simulink model "IEEE_9bus_new_o"  (R2024a)
settings: Solver=ode45  StartTime=0.0  StopTime=60/60  RelTol=1e-3  EnableMultiTasking=on
PreLoadFcn:
  | faultType = "ABCG";
  | faultLineStr = "Line 7-8";
  | faultDistance = 50;
  | L78_Length = 50;
  | L89_Length = 50;
  | L96_Length = 50;
  | L64_Length = 50;
  | L45_Length = 50;
  | L57_Length = 50;
  | 
  | mdl = load('lineIdentificationModel.mat');
  | lineMdl = mdl.treeModel;
  | 
  | mdl = load('typeIdentificationModelV2.mat');
  | typeMdl = mdl.treeModel;
  | 
  | mdl = load('faultLocationModel.mat');
  | locationMdl = mdl.treeModel;
libraries: dspstat3 x36, simulink x24, spsThreePhasePISectionLineLib x12, spsThreePhaseVIMeasurementLib x12, spsLoadFlowBusLib x9, spsThreePhaseFaultLib x6, jailib x3, spsThreePhaseSourceLib x3, spsThreePhaseTransformerTwoWindingsLib x3, statsLibrary x3, spsThreePhaseBreakerLib x3, sps_lib x1
(part 2 of 3)

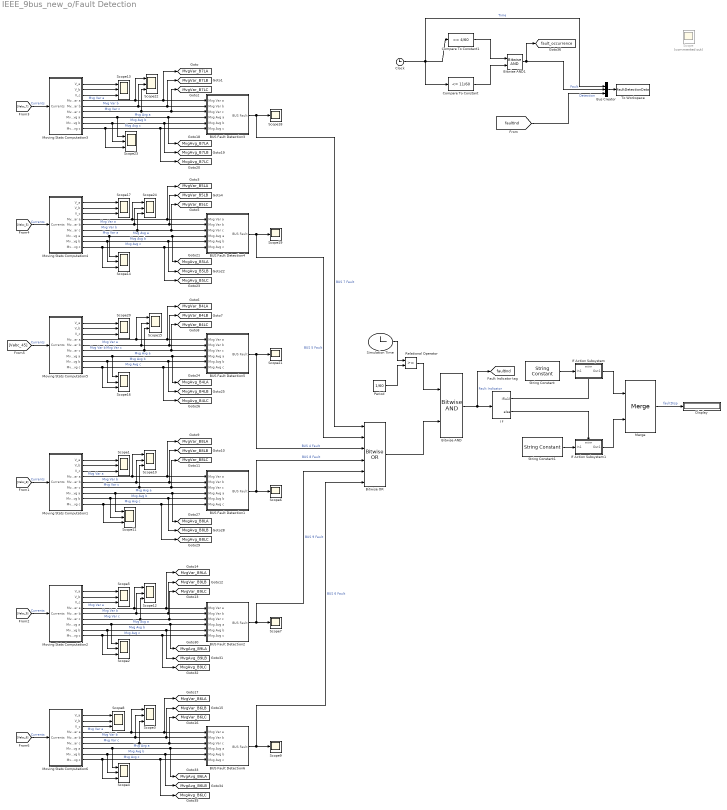
== system IEEE_9bus_new_o/Fault Detection ==
  BUS Fault Detection1 : Subsystem
  BUS Fault Detection2 : Subsystem
  BUS Fault Detection3 : Subsystem
  BUS Fault Detection4 : Subsystem
  BUS Fault Detection5 : Subsystem
  BUS Fault Detection6 : Subsystem
  Bitwise AND : simulink/Logic and Bit Operations/Bitwise Operator  logicop=AND  UseBitMask=off  NumInputPorts=2  BitMask=bin2dec('11011001')  BitMaskRealWorld=Stored Integer
      settings: LibrarySourceBlock=|
      | simulink/Quick Insert/Logic and Bit
      | Operations/Bitwise AND
  Bitwise AND1 : simulink/Logic and Bit Operations/Bitwise Operator  logicop=AND  UseBitMask=off  NumInputPorts=2  BitMask=bin2dec('11011001')  BitMaskRealWorld=Stored Integer
      settings: LibrarySourceBlock=|
      | simulink/Quick Insert/Logic and Bit
      | Operations/Bitwise AND
  Bitwise OR : simulink/Logic and Bit Operations/Bitwise Operator  logicop=OR  UseBitMask=off  NumInputPorts=6  BitMask=bin2dec('11011001')  BitMaskRealWorld=Stored Integer
      settings: LibrarySourceBlock=|
      | simulink/Quick Insert/Logic and Bit
      | Operations/Bitwise OR
  Bus Creator : BusCreator  Inputs=3
  Clock : Clock
  Compare To Constant : simulink/Logic and Bit Operations/Compare To Constant  relop=<=  const=11/60  OutDataTypeStr=boolean
  Compare To Constant1 : simulink/Logic and Bit Operations/Compare To Constant  relop=>=  const=4/60  OutDataTypeStr=boolean
  Display : Display
  I f : If  IfExpression=u1
  If Action Subsystem : Subsystem  TreatAsAtomicUnit=on
  If Action Subsystem1 : Subsystem  TreatAsAtomicUnit=on
  Merge : Merge
  Moving Stats Computation1 : Subsystem
  Moving Stats Computation2 : Subsystem
  Moving Stats Computation3 : Subsystem
  Moving Stats Computation4 : Subsystem
  Moving Stats Computation5 : Subsystem
  Moving Stats Computation6 : Subsystem
  Period : Constant  Value=1/60
  Relational Operator : RelationalOperator  OutDataTypeStr=boolean  RndMeth=Simplest  InputSameDT=off
  Scope : Scope  Commented=on  NumInputPorts=2
  Scope{1..5,8,10..17,20,22..24} (18 alike) : Scope  NumInputPorts=3
  Scope{6..7,9,18..19,21} (6 alike) : Scope
  Simulation Time : Clock
  String Constant : StringConstant  String="\"Faulted\""
  String Constant1 : StringConstant  String="\"\""
  To Workspace : ToWorkspace  VariableName=faultDetectionData  SaveFormat=Timeseries  SampleTime=-1
  tag scope: MvgAvg_B4LA=global, MvgAvg_B4LB=global, MvgAvg_B4LC=global, MvgAvg_B5LA=global, MvgAvg_B5LB=global, MvgAvg_B5LC=global, MvgAvg_B6LA=global, MvgAvg_B6LB=global, MvgAvg_B6LC=global, MvgAvg_B7LA=global, MvgAvg_B7LB=global, MvgAvg_B7LC=global, MvgAvg_B8LA=global, MvgAvg_B8LB=global, MvgAvg_B8LC=global, MvgAvg_B9LA=global, MvgAvg_B9LB=global, MvgAvg_B9LC=global, MvgVar_B4LA=global, MvgVar_B4LB=global, MvgVar_B4LC=global, MvgVar_B5LA=global, MvgVar_B5LB=global, MvgVar_B5LC=global, MvgVar_B6LA=global, MvgVar_B6LB=global, MvgVar_B6LC=global, MvgVar_B7LA=global, MvgVar_B7LB=global, MvgVar_B7LC=global, MvgVar_B8LA=global, MvgVar_B8LB=global, MvgVar_B8LC=global, MvgVar_B9LA=global, MvgVar_B9LB=global, MvgVar_B9LC=global, faultInd=global, fault_occurrence=global
  wires:
  BUS Fault Detection5/1(BUS Fault) -> Bitwise OR/3, Scope21/1  "BUS 4 Fault"
  BUS Fault Detection3/1(BUS Fault) -> Scope18/1, Bitwise OR/1  "BUS 7 Fault"
  Moving Stats Computation2/3(V_c) -> Scope5/3
  Moving Stats Computation6/5(Mvg Var b) -> BUS Fault Detection6/2(Mvg Var b), [MvgVar_B6LB], Scope3/2  "Mvg Var b"
  Moving Stats Computation6/7(Mvg Avg a) -> BUS Fault Detection6/4(Mvg Avg a), [MvgAvg_B6LA], Scope4/1  "Mvg Avg a"
  Moving Stats Computation3/6(Mvg Var c) -> BUS Fault Detection3/3(Mvg Var c), [MvgVar_B7LC], Scope22/3  "Mvg Var c"
  BUS Fault Detection6/1(BUS Fault) -> Bitwise OR/6, Scope9/1  "BUS 6 Fault"
  Moving Stats Computation1/8(Mvg Avg b) -> BUS Fault Detection1/5(Mvg Avg b), [MvgAvg_B8LB], Scope11/2  "Mvg Avg b"
  Moving Stats Computation5/4(Mvg Var a) -> BUS Fault Detection5/1(Mvg Var a), [MvgVar_B4LA], Scope15/1  "Mvg Var a"
  Moving Stats Computation1/5(Mvg Var b) -> BUS Fault Detection1/2(Mvg Var b), [MvgVar_B8LB], Scope10/2  "Mvg Var b"
  [Vabc_9] -> Moving Stats Computation2/1(Currents)  "Currents"
  Moving Stats Computation4/9(Mvg Avg c) -> BUS Fault Detection4/6(Mvg Avg c), [MvgAvg_B5LC], Scope14/3  "Mvg Avg c"
  Moving Stats Computation3/5(Mvg Var b) -> [MvgVar_B7LB], BUS Fault Detection3/2(Mvg Var b), Scope22/2  "Mvg Var b"
  Moving Stats Computation1/2(V_b) -> Scope1/2
  Moving Stats Computation1/7(Mvg Avg a) -> BUS Fault Detection1/4(Mvg Avg a), [MvgAvg_B8LA], Scope11/1  "Mvg Avg a"
  [Vabc_7] -> Moving Stats Computation3/1(Currents)  "Currents"
  Moving Stats Computation5/6(Mvg Var c) -> BUS Fault Detection5/3(Mvg Var c), [MvgVar_B4LC], Scope15/3  "Mvg Var c"
  Moving Stats Computation2/7(Mvg Avg a) -> BUS Fault Detection2/4(Mvg Avg a), [MvgAvg_B9LA], Scope2/1  "Mvg Avg a"
  Moving Stats Computation5/9(Mvg Avg c) -> BUS Fault Detection5/6(Mvg Avg c), [MvgAvg_B4LC], Scope16/3  "Mvg Avg c"
  Moving Stats Computation2/2(V_b) -> Scope5/2
  Moving Stats Computation4/1(V_a) -> Scope17/1
  Moving Stats Computation5/2(V_b) -> Scope20/2
  Moving Stats Computation3/1(V_a) -> Scope13/1
  Moving Stats Computation5/7(Mvg Avg a) -> BUS Fault Detection5/4(Mvg Avg a), [MvgAvg_B4LA], Scope16/1  "Mvg Avg a"
  [Vabc_8] -> Moving Stats Computation1/1(Currents)  "Currents"
  Moving Stats Computation6/2(V_b) -> Scope8/2
  Moving Stats Computation5/5(Mvg Var b) -> BUS Fault Detection5/2(Mvg Var b), [MvgVar_B4LB], Scope15/2  "Mvg Var b"
  Moving Stats Computation1/1(V_a) -> Scope1/1
  Moving Stats Computation5/8(Mvg Avg b) -> BUS Fault Detection5/5(Mvg Avg b), [MvgAvg_B4LB], Scope16/2  "Mvg Avg b"
  Moving Stats Computation2/1(V_a) -> Scope5/1
  Moving Stats Computation4/8(Mvg Avg b) -> BUS Fault Detection4/5(Mvg Avg b), [MvgAvg_B5LB], Scope14/2  "Mvg Avg b"
  BUS Fault Detection4/1(BUS Fault) -> Scope19/1, Bitwise OR/2  "BUS 5 Fault"
  BUS Fault Detection1/1(BUS Fault) -> Scope6/1, Bitwise OR/4  "BUS 8 Fault"
  Moving Stats Computation6/9(Mvg Avg c) -> BUS Fault Detection6/6(Mvg Avg c), [MvgAvg_B6LC], Scope4/3  "Mvg Avg c"
  Moving Stats Computation3/9(Mvg Avg c) -> [MvgAvg_B7LC], BUS Fault Detection3/6(Mvg Avg c), Scope23/3  "Mvg Avg c"
  Moving Stats Computation4/3(V_c) -> Scope17/3
  [Vabc_5] -> Moving Stats Computation4/1(Currents)  "Currents"
  Moving Stats Computation6/1(V_a) -> Scope8/1
  Moving Stats Computation5/1(V_a) -> Scope20/1
  Moving Stats Computation1/3(V_c) -> Scope1/3
  Moving Stats Computation2/5(Mvg Var b) -> BUS Fault Detection2/2(Mvg Var b), [MvgVar_B9LB], Scope12/2  "Mvg Var b"
  Moving Stats Computation5/3(V_c) -> Scope20/3
  Moving Stats Computation6/3(V_c) -> Scope8/3
  Moving Stats Computation3/8(Mvg Avg b) -> [MvgAvg_B7LB], BUS Fault Detection3/5(Mvg Avg b), Scope23/2  "Mvg Avg b"
  [Vabc_45] -> Moving Stats Computation5/1(Currents)  "Currents"
  Moving Stats Computation3/3(V_c) -> Scope13/3
  Moving Stats Computation6/8(Mvg Avg b) -> BUS Fault Detection6/5(Mvg Avg b), [MvgAvg_B6LB], Scope4/2  "Mvg Avg b"
  Moving Stats Computation4/7(Mvg Avg a) -> BUS Fault Detection4/4(Mvg Avg a), [MvgAvg_B5LA], Scope14/1  "Mvg Avg a"
  Moving Stats Computation3/7(Mvg Avg a) -> BUS Fault Detection3/4(Mvg Avg a), [MvgAvg_B7LA], Scope23/1  "Mvg Avg a"
  Moving Stats Computation3/4(Mvg Var a) -> [MvgVar_B7LA], BUS Fault Detection3/1(Mvg Var a), Scope22/1  "Mvg Var a"
  Moving Stats Computation2/6(Mvg Var c) -> BUS Fault Detection2/3(Mvg Var c), [MvgVar_B9LC], Scope12/3  "Mvg Var c"
  Moving Stats Computation3/2(V_b) -> Scope13/2
  Moving Stats Computation2/9(Mvg Avg c) -> BUS Fault Detection2/6(Mvg Avg c), [MvgAvg_B9LC], Scope2/3  "Mvg Avg c"
  Moving Stats Computation4/2(V_b) -> Scope17/2
  Moving Stats Computation6/6(Mvg Var c) -> BUS Fault Detection6/3(Mvg Var c), [MvgVar_B6LC], Scope3/3  "Mvg Var c"
  Moving Stats Computation6/4(Mvg Var a) -> BUS Fault Detection6/1(Mvg Var a), [MvgVar_B6LA], Scope3/1  "Mvg Var a"
  BUS Fault Detection2/1(BUS Fault) -> Scope7/1, Bitwise OR/5  "BUS 9 Fault"
  Moving Stats Computation2/8(Mvg Avg b) -> BUS Fault Detection2/5(Mvg Avg b), [MvgAvg_B9LB], Scope2/2  "Mvg Avg b"
  Moving Stats Computation2/4(Mvg Var a) -> BUS Fault Detection2/1(Mvg Var a), [MvgVar_B9LA], Scope12/1  "Mvg Var a"
  [Vabc_6] -> Moving Stats Computation6/1(Currents)  "Currents"
  Moving Stats Computation1/9(Mvg Avg c) -> BUS Fault Detection1/6(Mvg Avg c), [MvgAvg_B8LC], Scope11/3  "Mvg Avg c"
  Moving Stats Computation1/4(Mvg Var a) -> BUS Fault Detection1/1(Mvg Var a), [MvgVar_B8LA], Scope10/1  "Mvg Var a"
  Moving Stats Computation1/6(Mvg Var c) -> BUS Fault Detection1/3(Mvg Var c), [MvgVar_B8LC], Scope10/3  "Mvg Var c"
  Simulation Time/1 -> Relational Operator/1
  Period/1 -> Relational Operator/2
  Relational Operator/1 -> Bitwise AND/1
  Bitwise OR/1 -> Bitwise AND/2
  Bitwise AND/1 -> [faultInd], I f/1  "Fault Indicator"
  I f/1 -> If Action Subsystem/Action
  I f/2 -> If Action Subsystem1/Action
  String Constant/1 -> If Action Subsystem/1(In1)
  String Constant1/1 -> If Action Subsystem1/1(In1)
  If Action Subsystem/1(Out1) -> Merge/1
  If Action Subsystem1/1(Out1) -> Merge/2
  Moving Stats Computation4/4(Mvg Var a) -> BUS Fault Detection4/1(Mvg Var a), [MvgVar_B5LA], Scope24/1  "Mvg Var a"
  Moving Stats Computation4/5(Mvg Var b) -> BUS Fault Detection4/2(Mvg Var b), [MvgVar_B5LB], Scope24/2  "Mvg Var b"
  Moving Stats Computation4/6(Mvg Var c) -> BUS Fault Detection4/3(Mvg Var c), [MvgVar_B5LC], Scope24/3  "Mvg Var a"
  Merge/1 -> Display/1  "faultDisp"
  Clock/1 -> Bus Creator/1, Compare To Constant1/1, Compare To Constant/1  "Time"
  Compare To Constant1/1 -> Bitwise AND1/1
  Compare To Constant/1 -> Bitwise AND1/2
  Bitwise AND1/1 -> Bus Creator/2, [fault_occurrence]  "Fault"
  [faultInd] -> Bus Creator/3  "Detection"
  Bus Creator/1 -> To Workspace/1

== system IEEE_9bus_new_o/Fault Line Identification ==
  Display : Display
  Fault Line Prediction : statsLibrary/Classification/ClassificationTree Predict  TrainedLearner=lineMdl  ShowOutputScore=off  LabelOutMin=[]  LabelOutMax=[]  ScoreOutMin=[]  ScoreOutMax=[]  RawScoreOutMin=[]  RawScoreOutMax=[]  StoredEnumName=lineMdl_enumLabels
  If : If  IfExpression=u1~=0
  If Action Subsystem : Subsystem  TreatAsAtomicUnit=on
  If Action Subsystem1 : Subsystem  TreatAsAtomicUnit=on
  Merge : Merge
  String Constant : StringConstant  String="\"\""
  To String : ToString
  wires:
  If Action Subsystem/1(Out1) -> Merge/1
  String Constant/1 -> If Action Subsystem1/1(In1)
  If/2 -> If Action Subsystem1/Action
  If Action Subsystem1/1(Out1) -> Merge/2
  To String/1 -> If Action Subsystem/1(In1)
  [faultInd] -> If/1
  [MvgStats] -> Fault Line Prediction/1
  Fault Line Prediction/1 -> To String/1
  If/1 -> If Action Subsystem/Action
  Merge/1 -> Display/1  "LineDisp"

== system IEEE_9bus_new_o/Fault Location ==
  Display : Display
  Fault Location Prediction : statsLibrary/Regression/RegressionTree Predict  TrainedLearner=locationMdl  OutMin=[]  OutMax=[]
  If : If  IfExpression=u1~=0
  If Action Subsystem : Subsystem  TreatAsAtomicUnit=on
  If Action Subsystem1 : Subsystem  TreatAsAtomicUnit=on
  Merge : Merge
  String Constant : StringConstant  String="\"\""
  To String : ToString
  wires:
  If Action Subsystem/1(Out1) -> Merge/1
  String Constant/1 -> If Action Subsystem1/1(In1)
  If/2 -> If Action Subsystem1/Action
  If Action Subsystem1/1(Out1) -> Merge/2
  To String/1 -> If Action Subsystem/1(In1)
  [faultInd] -> If/1
  [MvgStats] -> Fault Location Prediction/1
  Fault Location Prediction/1 -> To String/1
  If/1 -> If Action Subsystem/Action
  Merge/1 -> Display/1  "LocationDisp"

== system IEEE_9bus_new_o/Fault Type Identification ==
  Display : Display
  Fault Type Prediction : statsLibrary/Classification/ClassificationTree Predict  TrainedLearner=typeMdl  ShowOutputScore=off  LabelOutMin=[]  LabelOutMax=[]  ScoreOutMin=[]  ScoreOutMax=[]  RawScoreOutMin=[]  RawScoreOutMax=[]  StoredEnumName=typeMdl_enumLabels
  If : If  IfExpression=u1~=0
  If Action Subsystem : Subsystem  TreatAsAtomicUnit=on
  If Action Subsystem1 : Subsystem  TreatAsAtomicUnit=on
  Merge : Merge
  String Constant : StringConstant  String="\"\""
  To String : ToString
  wires:
  If/1 -> If Action Subsystem/Action
  Fault Type Prediction/1 -> To String/1
  [MvgStats] -> Fault Type Prediction/1
  [faultInd] -> If/1
  To String/1 -> If Action Subsystem/1(In1)
  If Action Subsystem1/1(Out1) -> Merge/2
  If/2 -> If Action Subsystem1/Action
  String Constant/1 -> If Action Subsystem1/1(In1)
  If Action Subsystem/1(Out1) -> Merge/1
  Merge/1 -> Display/1  "TypeDisp"

== system IEEE_9bus_new_o/Relay System ==
  Bitwise AND2 : simulink/Logic and Bit Operations/Bitwise Operator  logicop=AND  UseBitMask=off  NumInputPorts=10  BitMask=bin2dec('11011001')  BitMaskRealWorld=Stored Integer
      settings: LibrarySourceBlock=|
      | simulink/Quick Insert/Logic and Bit
      | Operations/Bitwise AND
  Delay : Delay  DelayLength=1
  Delay1 : Delay  DelayLength=3
  Delay2 : Delay  DelayLength=4
  Delay3 : Delay  DelayLength=5
  Delay4 : Delay  DelayLength=6
  Delay5 : Delay  DelayLength=7
  Delay6 : Delay  DelayLength=8
  Delay7 : Delay  DelayLength=9
  Delay8 : Delay  DelayLength=10
  Delay9 : Delay  DelayLength=10
  Scope : Scope  NumInputPorts=3
  tag scope: tripInd=global
  wires:
  Bitwise AND2/1 -> Scope/3, [tripInd]  "Relay Activation"
  [faultInd] -> Scope/2, Delay/1, Delay1/1, Delay2/1, Delay3/1, Delay4/1, Delay5/1, Delay6/1, Delay7/1, Delay9/1, Delay8/1  "Detection"
  Delay4/1 -> Bitwise AND2/5
  Delay1/1 -> Bitwise AND2/2
  Delay9/1 -> Bitwise AND2/10
  Delay5/1 -> Bitwise AND2/6
  Delay3/1 -> Bitwise AND2/4
  Delay8/1 -> Bitwise AND2/9
  Delay6/1 -> Bitwise AND2/7
  Delay2/1 -> Bitwise AND2/3
  Delay/1 -> Bitwise AND2/1
  Delay7/1 -> Bitwise AND2/8
  [fault_occurrence] -> Scope/1  "Fault"

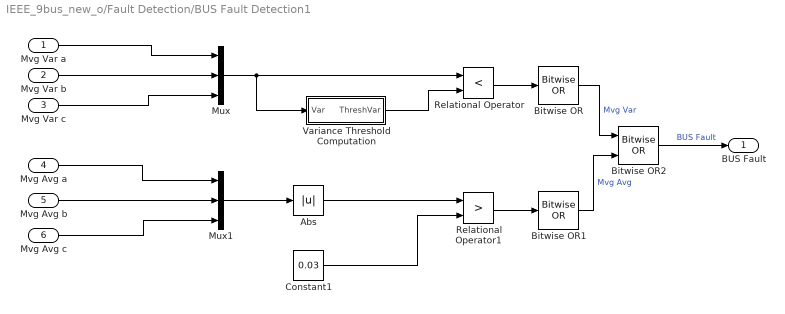
== system IEEE_9bus_new_o/Fault Detection/BUS Fault Detection1 ==
  Mvg Var a : Inport
  Mvg Var b : Inport  Port=2
  Mvg Var c : Inport  Port=3
  Mvg Avg a : Inport  Port=4
  Mvg Avg b : Inport  Port=5
  Mvg Avg c : Inport  Port=6
  Abs : Abs  SaturateOnIntegerOverflow=off
  Bitwise OR : simulink/Logic and Bit Operations/Bitwise Operator  logicop=OR  UseBitMask=off  BitMask=bin2dec('11011001')  BitMaskRealWorld=Stored Integer
      settings: LibrarySourceBlock=|
      | simulink/Quick Insert/Logic and Bit
      | Operations/Bitwise OR
  Bitwise OR1 : simulink/Logic and Bit Operations/Bitwise Operator  logicop=OR  UseBitMask=off  BitMask=bin2dec('11011001')  BitMaskRealWorld=Stored Integer
      settings: LibrarySourceBlock=|
      | simulink/Quick Insert/Logic and Bit
      | Operations/Bitwise OR
  Bitwise OR2 : simulink/Logic and Bit Operations/Bitwise Operator  logicop=OR  UseBitMask=off  NumInputPorts=2  BitMask=bin2dec('11011001')  BitMaskRealWorld=Stored Integer
      settings: LibrarySourceBlock=|
      | simulink/Quick Insert/Logic and Bit
      | Operations/Bitwise OR
  Constant1 : Constant  Value=0.03
  Mux : Mux  Inputs=3
  Mux1 : Mux  Inputs=3
  Relational Operator : RelationalOperator  Operator=<  OutDataTypeStr=boolean  RndMeth=Simplest  InputSameDT=off
  Relational Operator1 : RelationalOperator  Operator=>  OutDataTypeStr=boolean  RndMeth=Simplest  InputSameDT=off
  Variance Threshold Computation : Subsystem
  BUS Fault : Outport
  wires:
  Variance Threshold Computation/1(ThreshVar) -> Relational Operator/2
  Mvg Var b/1 -> Mux/2
  Abs/1 -> Relational Operator1/1
  Constant1/1 -> Relational Operator1/2
  Bitwise OR/1 -> Bitwise OR2/1  "Mvg Var"
  Bitwise OR1/1 -> Bitwise OR2/2  "Mvg Avg"
  Mux/1 -> Relational Operator/1, Variance Threshold Computation/1(Var)
  Relational Operator/1 -> Bitwise OR/1
  Bitwise OR2/1 -> BUS Fault/1  "BUS Fault"
  Relational Operator1/1 -> Bitwise OR1/1
  Mux1/1 -> Abs/1
  Mvg Avg a/1 -> Mux1/1
  Mvg Avg c/1 -> Mux1/3
  Mvg Var a/1 -> Mux/1
  Mvg Var c/1 -> Mux/3
  Mvg Avg b/1 -> Mux1/2

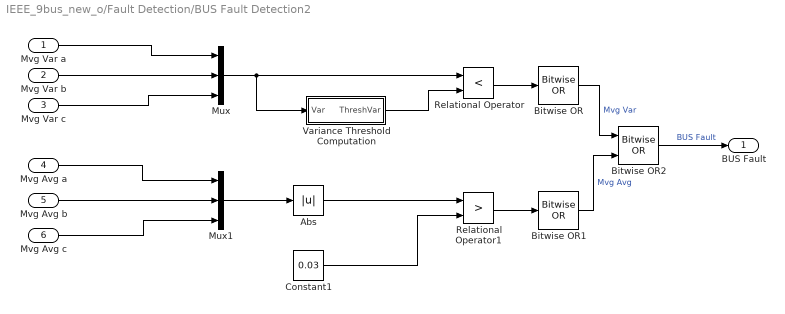
== system IEEE_9bus_new_o/Fault Detection/BUS Fault Detection2 ==
  Mvg Var a : Inport
  Mvg Var b : Inport  Port=2
  Mvg Var c : Inport  Port=3
  Mvg Avg a : Inport  Port=4
  Mvg Avg b : Inport  Port=5
  Mvg Avg c : Inport  Port=6
  Abs : Abs  SaturateOnIntegerOverflow=off
  Bitwise OR : simulink/Logic and Bit Operations/Bitwise Operator  logicop=OR  UseBitMask=off  BitMask=bin2dec('11011001')  BitMaskRealWorld=Stored Integer
      settings: LibrarySourceBlock=|
      | simulink/Quick Insert/Logic and Bit
      | Operations/Bitwise OR
  Bitwise OR1 : simulink/Logic and Bit Operations/Bitwise Operator  logicop=OR  UseBitMask=off  BitMask=bin2dec('11011001')  BitMaskRealWorld=Stored Integer
      settings: LibrarySourceBlock=|
      | simulink/Quick Insert/Logic and Bit
      | Operations/Bitwise OR
  Bitwise OR2 : simulink/Logic and Bit Operations/Bitwise Operator  logicop=OR  UseBitMask=off  NumInputPorts=2  BitMask=bin2dec('11011001')  BitMaskRealWorld=Stored Integer
      settings: LibrarySourceBlock=|
      | simulink/Quick Insert/Logic and Bit
      | Operations/Bitwise OR
  Constant1 : Constant  Value=0.03
  Mux : Mux  Inputs=3
  Mux1 : Mux  Inputs=3
  Relational Operator : RelationalOperator  Operator=<  OutDataTypeStr=boolean  RndMeth=Simplest  InputSameDT=off
  Relational Operator1 : RelationalOperator  Operator=>  OutDataTypeStr=boolean  RndMeth=Simplest  InputSameDT=off
  Variance Threshold Computation : Subsystem
  BUS Fault : Outport
  wires:
  Mvg Avg b/1 -> Mux1/2
  Mvg Var c/1 -> Mux/3
  Mvg Var a/1 -> Mux/1
  Mvg Avg c/1 -> Mux1/3
  Mvg Avg a/1 -> Mux1/1
  Mux1/1 -> Abs/1
  Relational Operator1/1 -> Bitwise OR1/1
  Bitwise OR2/1 -> BUS Fault/1  "BUS Fault"
  Relational Operator/1 -> Bitwise OR/1
  Mux/1 -> Variance Threshold Computation/1(Var), Relational Operator/1
  Bitwise OR1/1 -> Bitwise OR2/2  "Mvg Avg"
  Bitwise OR/1 -> Bitwise OR2/1  "Mvg Var"
  Constant1/1 -> Relational Operator1/2
  Abs/1 -> Relational Operator1/1
  Mvg Var b/1 -> Mux/2
  Variance Threshold Computation/1(ThreshVar) -> Relational Operator/2

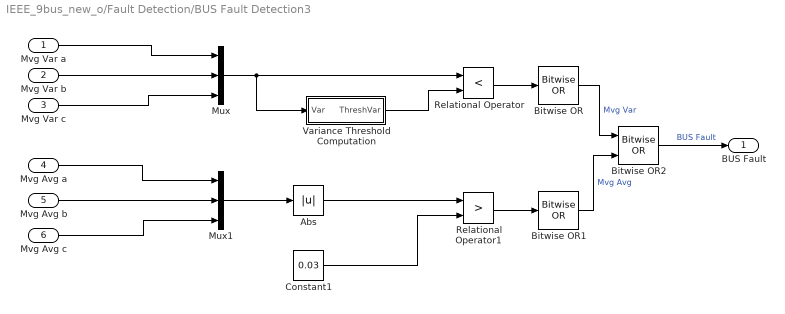
== system IEEE_9bus_new_o/Fault Detection/BUS Fault Detection3 ==
  Mvg Var a : Inport
  Mvg Var b : Inport  Port=2
  Mvg Var c : Inport  Port=3
  Mvg Avg a : Inport  Port=4
  Mvg Avg b : Inport  Port=5
  Mvg Avg c : Inport  Port=6
  Abs : Abs  SaturateOnIntegerOverflow=off
  Bitwise OR : simulink/Logic and Bit Operations/Bitwise Operator  logicop=OR  UseBitMask=off  BitMask=bin2dec('11011001')  BitMaskRealWorld=Stored Integer
      settings: LibrarySourceBlock=|
      | simulink/Quick Insert/Logic and Bit
      | Operations/Bitwise OR
  Bitwise OR1 : simulink/Logic and Bit Operations/Bitwise Operator  logicop=OR  UseBitMask=off  BitMask=bin2dec('11011001')  BitMaskRealWorld=Stored Integer
      settings: LibrarySourceBlock=|
      | simulink/Quick Insert/Logic and Bit
      | Operations/Bitwise OR
  Bitwise OR2 : simulink/Logic and Bit Operations/Bitwise Operator  logicop=OR  UseBitMask=off  NumInputPorts=2  BitMask=bin2dec('11011001')  BitMaskRealWorld=Stored Integer
      settings: LibrarySourceBlock=|
      | simulink/Quick Insert/Logic and Bit
      | Operations/Bitwise OR
  Constant1 : Constant  Value=0.03
  Mux : Mux  Inputs=3
  Mux1 : Mux  Inputs=3
  Relational Operator : RelationalOperator  Operator=<  OutDataTypeStr=boolean  RndMeth=Simplest  InputSameDT=off
  Relational Operator1 : RelationalOperator  Operator=>  OutDataTypeStr=boolean  RndMeth=Simplest  InputSameDT=off
  Variance Threshold Computation : Subsystem
  BUS Fault : Outport
  wires:
  Mvg Avg b/1 -> Mux1/2
  Mvg Var c/1 -> Mux/3
  Mvg Var a/1 -> Mux/1
  Mvg Avg c/1 -> Mux1/3
  Mvg Avg a/1 -> Mux1/1
  Mux1/1 -> Abs/1
  Relational Operator1/1 -> Bitwise OR1/1
  Bitwise OR2/1 -> BUS Fault/1  "BUS Fault"
  Relational Operator/1 -> Bitwise OR/1
  Mux/1 -> Variance Threshold Computation/1(Var), Relational Operator/1
  Bitwise OR1/1 -> Bitwise OR2/2  "Mvg Avg"
  Bitwise OR/1 -> Bitwise OR2/1  "Mvg Var"
  Constant1/1 -> Relational Operator1/2
  Abs/1 -> Relational Operator1/1
  Mvg Var b/1 -> Mux/2
  Variance Threshold Computation/1(ThreshVar) -> Relational Operator/2

== system IEEE_9bus_new_o/Fault Detection/BUS Fault Detection4 ==
  Mvg Var a : Inport
  Mvg Var b : Inport  Port=2
  Mvg Var c : Inport  Port=3
  Mvg Avg a : Inport  Port=4
  Mvg Avg b : Inport  Port=5
  Mvg Avg c : Inport  Port=6
  Abs : Abs  SaturateOnIntegerOverflow=off
  Bitwise OR : simulink/Logic and Bit Operations/Bitwise Operator  logicop=OR  UseBitMask=off  BitMask=bin2dec('11011001')  BitMaskRealWorld=Stored Integer
      settings: LibrarySourceBlock=|
      | simulink/Quick Insert/Logic and Bit
      | Operations/Bitwise OR
  Bitwise OR1 : simulink/Logic and Bit Operations/Bitwise Operator  logicop=OR  UseBitMask=off  BitMask=bin2dec('11011001')  BitMaskRealWorld=Stored Integer
      settings: LibrarySourceBlock=|
      | simulink/Quick Insert/Logic and Bit
      | Operations/Bitwise OR
  Bitwise OR2 : simulink/Logic and Bit Operations/Bitwise Operator  logicop=OR  UseBitMask=off  NumInputPorts=2  BitMask=bin2dec('11011001')  BitMaskRealWorld=Stored Integer
      settings: LibrarySourceBlock=|
      | simulink/Quick Insert/Logic and Bit
      | Operations/Bitwise OR
  Constant1 : Constant  Value=0.03
  Mux : Mux  Inputs=3
  Mux1 : Mux  Inputs=3
  Relational Operator : RelationalOperator  Operator=<  OutDataTypeStr=boolean  RndMeth=Simplest  InputSameDT=off
  Relational Operator1 : RelationalOperator  Operator=>  OutDataTypeStr=boolean  RndMeth=Simplest  InputSameDT=off
  Variance Threshold Computation : Subsystem
  BUS Fault : Outport
  wires:
  Variance Threshold Computation/1(ThreshVar) -> Relational Operator/2
  Mvg Var b/1 -> Mux/2
  Abs/1 -> Relational Operator1/1
  Constant1/1 -> Relational Operator1/2
  Bitwise OR/1 -> Bitwise OR2/1  "Mvg Var"
  Bitwise OR1/1 -> Bitwise OR2/2  "Mvg Avg"
  Mux/1 -> Relational Operator/1, Variance Threshold Computation/1(Var)
  Relational Operator/1 -> Bitwise OR/1
  Bitwise OR2/1 -> BUS Fault/1  "BUS Fault"
  Relational Operator1/1 -> Bitwise OR1/1
  Mux1/1 -> Abs/1
  Mvg Avg a/1 -> Mux1/1
  Mvg Avg c/1 -> Mux1/3
  Mvg Var a/1 -> Mux/1
  Mvg Var c/1 -> Mux/3
  Mvg Avg b/1 -> Mux1/2

== system IEEE_9bus_new_o/Fault Detection/BUS Fault Detection5 ==
  Mvg Var a : Inport
  Mvg Var b : Inport  Port=2
  Mvg Var c : Inport  Port=3
  Mvg Avg a : Inport  Port=4
  Mvg Avg b : Inport  Port=5
  Mvg Avg c : Inport  Port=6
  Abs : Abs  SaturateOnIntegerOverflow=off
  Bitwise OR : simulink/Logic and Bit Operations/Bitwise Operator  logicop=OR  UseBitMask=off  BitMask=bin2dec('11011001')  BitMaskRealWorld=Stored Integer
      settings: LibrarySourceBlock=|
      | simulink/Quick Insert/Logic and Bit
      | Operations/Bitwise OR
  Bitwise OR1 : simulink/Logic and Bit Operations/Bitwise Operator  logicop=OR  UseBitMask=off  BitMask=bin2dec('11011001')  BitMaskRealWorld=Stored Integer
      settings: LibrarySourceBlock=|
      | simulink/Quick Insert/Logic and Bit
      | Operations/Bitwise OR
  Bitwise OR2 : simulink/Logic and Bit Operations/Bitwise Operator  logicop=OR  UseBitMask=off  NumInputPorts=2  BitMask=bin2dec('11011001')  BitMaskRealWorld=Stored Integer
      settings: LibrarySourceBlock=|
      | simulink/Quick Insert/Logic and Bit
      | Operations/Bitwise OR
  Constant1 : Constant  Value=0.03
  Mux : Mux  Inputs=3
  Mux1 : Mux  Inputs=3
  Relational Operator : RelationalOperator  Operator=<  OutDataTypeStr=boolean  RndMeth=Simplest  InputSameDT=off
  Relational Operator1 : RelationalOperator  Operator=>  OutDataTypeStr=boolean  RndMeth=Simplest  InputSameDT=off
  Variance Threshold Computation : Subsystem
  BUS Fault : Outport
  wires:
  Mvg Avg b/1 -> Mux1/2
  Mvg Var c/1 -> Mux/3
  Mvg Var a/1 -> Mux/1
  Mvg Avg c/1 -> Mux1/3
  Mvg Avg a/1 -> Mux1/1
  Mux1/1 -> Abs/1
  Relational Operator1/1 -> Bitwise OR1/1
  Bitwise OR2/1 -> BUS Fault/1  "BUS Fault"
  Relational Operator/1 -> Bitwise OR/1
  Mux/1 -> Variance Threshold Computation/1(Var), Relational Operator/1
  Bitwise OR1/1 -> Bitwise OR2/2  "Mvg Avg"
  Bitwise OR/1 -> Bitwise OR2/1  "Mvg Var"
  Constant1/1 -> Relational Operator1/2
  Abs/1 -> Relational Operator1/1
  Mvg Var b/1 -> Mux/2
  Variance Threshold Computation/1(ThreshVar) -> Relational Operator/2

== system IEEE_9bus_new_o/Fault Detection/BUS Fault Detection6 ==
  Mvg Var a : Inport
  Mvg Var b : Inport  Port=2
  Mvg Var c : Inport  Port=3
  Mvg Avg a : Inport  Port=4
  Mvg Avg b : Inport  Port=5
  Mvg Avg c : Inport  Port=6
  Abs : Abs  SaturateOnIntegerOverflow=off
  Bitwise OR : simulink/Logic and Bit Operations/Bitwise Operator  logicop=OR  UseBitMask=off  BitMask=bin2dec('11011001')  BitMaskRealWorld=Stored Integer
      settings: LibrarySourceBlock=|
      | simulink/Quick Insert/Logic and Bit
      | Operations/Bitwise OR
  Bitwise OR1 : simulink/Logic and Bit Operations/Bitwise Operator  logicop=OR  UseBitMask=off  BitMask=bin2dec('11011001')  BitMaskRealWorld=Stored Integer
      settings: LibrarySourceBlock=|
      | simulink/Quick Insert/Logic and Bit
      | Operations/Bitwise OR
  Bitwise OR2 : simulink/Logic and Bit Operations/Bitwise Operator  logicop=OR  UseBitMask=off  NumInputPorts=2  BitMask=bin2dec('11011001')  BitMaskRealWorld=Stored Integer
      settings: LibrarySourceBlock=|
      | simulink/Quick Insert/Logic and Bit
      | Operations/Bitwise OR
  Constant1 : Constant  Value=0.03
  Mux : Mux  Inputs=3
  Mux1 : Mux  Inputs=3
  Relational Operator : RelationalOperator  Operator=<  OutDataTypeStr=boolean  RndMeth=Simplest  InputSameDT=off
  Relational Operator1 : RelationalOperator  Operator=>  OutDataTypeStr=boolean  RndMeth=Simplest  InputSameDT=off
  Variance Threshold Computation : Subsystem
  BUS Fault : Outport
  wires:
  Variance Threshold Computation/1(ThreshVar) -> Relational Operator/2
  Mvg Var b/1 -> Mux/2
  Abs/1 -> Relational Operator1/1
  Constant1/1 -> Relational Operator1/2
  Bitwise OR/1 -> Bitwise OR2/1  "Mvg Var"
  Bitwise OR1/1 -> Bitwise OR2/2  "Mvg Avg"
  Mux/1 -> Relational Operator/1, Variance Threshold Computation/1(Var)
  Relational Operator/1 -> Bitwise OR/1
  Bitwise OR2/1 -> BUS Fault/1  "BUS Fault"
  Relational Operator1/1 -> Bitwise OR1/1
  Mux1/1 -> Abs/1
  Mvg Avg a/1 -> Mux1/1
  Mvg Avg c/1 -> Mux1/3
  Mvg Var a/1 -> Mux/1
  Mvg Var c/1 -> Mux/3
  Mvg Avg b/1 -> Mux1/2

== system IEEE_9bus_new_o/Fault Detection/If Action Subsystem ==
  In1 : Inport
  Action Port : ActionPort  ActionPortLabel=if(u1)
  Out1 : Outport
  wires:
  In1/1 -> Out1/1

== system IEEE_9bus_new_o/Fault Detection/If Action Subsystem1 ==
  In1 : Inport
  Action Port : ActionPort  ActionPortLabel=else
  Out1 : Outport
  wires:
  In1/1 -> Out1/1

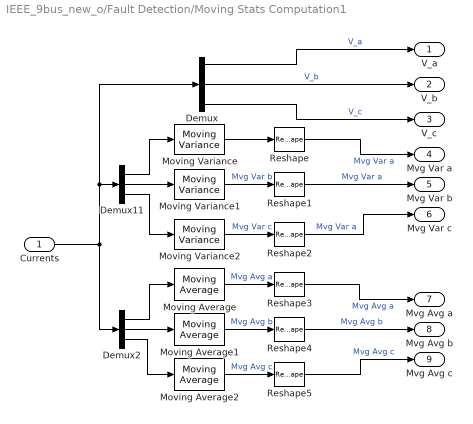
== system IEEE_9bus_new_o/Fault Detection/Moving Stats Computation1 ==
  Currents : Inport
  Demux : Demux  Outputs=3
  Demux11 : Demux  Outputs=3
  Demux2 : Demux  Outputs=3
  Moving Average : dspstat3/Moving Average  Method=Sliding window  ForgettingFactorPort=off  SpecifyWindowLength=on  WindowLength=100  OverlapLength=99  AllowArbitraryInputLength=off  ForgettingFactor=0.9  SimulateUsing=Interpreted execution
  Moving Average1 : dspstat3/Moving Average  Method=Sliding window  ForgettingFactorPort=off  SpecifyWindowLength=on  WindowLength=100  OverlapLength=99  AllowArbitraryInputLength=off  ForgettingFactor=0.9  SimulateUsing=Interpreted execution
  Moving Average2 : dspstat3/Moving Average  Method=Sliding window  ForgettingFactorPort=off  SpecifyWindowLength=on  WindowLength=100  OverlapLength=99  AllowArbitraryInputLength=off  ForgettingFactor=0.9  SimulateUsing=Interpreted execution
  Moving Variance : dspstat3/Moving Variance  Method=Sliding window  ForgettingFactorPort=off  SpecifyWindowLength=on  WindowLength=100  OverlapLength=99  AllowArbitraryInputLength=off  ForgettingFactor=0.9  SimulateUsing=Interpreted execution
  Moving Variance1 : dspstat3/Moving Variance  Method=Sliding window  ForgettingFactorPort=off  SpecifyWindowLength=on  WindowLength=100  OverlapLength=99  AllowArbitraryInputLength=off  ForgettingFactor=0.9  SimulateUsing=Interpreted execution
  Moving Variance2 : dspstat3/Moving Variance  Method=Sliding window  ForgettingFactorPort=off  SpecifyWindowLength=on  WindowLength=100  OverlapLength=99  AllowArbitraryInputLength=off  ForgettingFactor=0.9  SimulateUsing=Interpreted execution
  Reshape{,1..5} (6 alike) : Reshape  OutputDimensionality=Customize  OutputDimensions=1
  V_a : Outport
  V_b : Outport  Port=2
  V_c : Outport  Port=3
  Mvg Var a : Outport  Port=4
  Mvg Var b : Outport  Port=5
  Mvg Var c : Outport  Port=6
  Mvg Avg a : Outport  Port=7
  Mvg Avg b : Outport  Port=8
  Mvg Avg c : Outport  Port=9
  wires:
  Reshape5/1 -> Mvg Avg c/1  "Mvg Avg c"
  Reshape4/1 -> Mvg Avg b/1  "Mvg Avg b"
  Reshape3/1 -> Mvg Avg a/1  "Mvg Avg a"
  Reshape2/1 -> Mvg Var c/1  "Mvg Var a"
  Reshape1/1 -> Mvg Var b/1  "Mvg Var a"
  Moving Variance/1 -> Reshape/1
  Demux11/2 -> Moving Variance1/1
  Demux/2 -> V_b/1  "V_b"
  Demux2/1 -> Moving Average/1
  Moving Average1/1 -> Reshape4/1  "Mvg Avg b"
  Currents/1 -> Demux/1, Demux11/1, Demux2/1
  Demux11/1 -> Moving Variance/1
  Demux11/3 -> Moving Variance2/1
  Moving Average/1 -> Reshape3/1  "Mvg Avg a"
  Demux2/2 -> Moving Average1/1
  Demux2/3 -> Moving Average2/1
  Moving Average2/1 -> Reshape5/1  "Mvg Avg c"
  Reshape/1 -> Mvg Var a/1  "Mvg Var a"
  Moving Variance2/1 -> Reshape2/1  "Mvg Var c"
  Moving Variance1/1 -> Reshape1/1  "Mvg Var b"
  Demux/3 -> V_c/1  "V_c"
  Demux/1 -> V_a/1  "V_a"

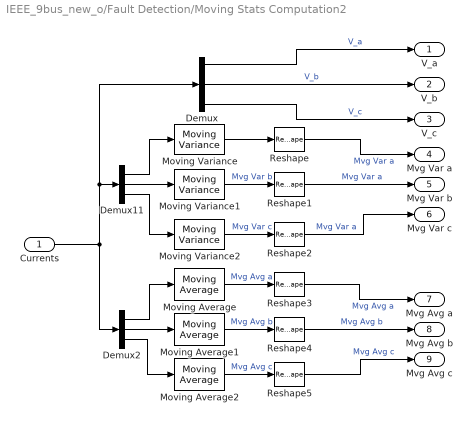
== system IEEE_9bus_new_o/Fault Detection/Moving Stats Computation2 ==
  Currents : Inport
  Demux : Demux  Outputs=3
  Demux11 : Demux  Outputs=3
  Demux2 : Demux  Outputs=3
  Moving Average : dspstat3/Moving Average  Method=Sliding window  ForgettingFactorPort=off  SpecifyWindowLength=on  WindowLength=100  OverlapLength=99  AllowArbitraryInputLength=off  ForgettingFactor=0.9  SimulateUsing=Interpreted execution
  Moving Average1 : dspstat3/Moving Average  Method=Sliding window  ForgettingFactorPort=off  SpecifyWindowLength=on  WindowLength=100  OverlapLength=99  AllowArbitraryInputLength=off  ForgettingFactor=0.9  SimulateUsing=Interpreted execution
  Moving Average2 : dspstat3/Moving Average  Method=Sliding window  ForgettingFactorPort=off  SpecifyWindowLength=on  WindowLength=100  OverlapLength=99  AllowArbitraryInputLength=off  ForgettingFactor=0.9  SimulateUsing=Interpreted execution
  Moving Variance : dspstat3/Moving Variance  Method=Sliding window  ForgettingFactorPort=off  SpecifyWindowLength=on  WindowLength=100  OverlapLength=99  AllowArbitraryInputLength=off  ForgettingFactor=0.9  SimulateUsing=Interpreted execution
  Moving Variance1 : dspstat3/Moving Variance  Method=Sliding window  ForgettingFactorPort=off  SpecifyWindowLength=on  WindowLength=100  OverlapLength=99  AllowArbitraryInputLength=off  ForgettingFactor=0.9  SimulateUsing=Interpreted execution
  Moving Variance2 : dspstat3/Moving Variance  Method=Sliding window  ForgettingFactorPort=off  SpecifyWindowLength=on  WindowLength=100  OverlapLength=99  AllowArbitraryInputLength=off  ForgettingFactor=0.9  SimulateUsing=Interpreted execution
  Reshape{,1..5} (6 alike) : Reshape  OutputDimensionality=Customize  OutputDimensions=1
  V_a : Outport
  V_b : Outport  Port=2
  V_c : Outport  Port=3
  Mvg Var a : Outport  Port=4
  Mvg Var b : Outport  Port=5
  Mvg Var c : Outport  Port=6
  Mvg Avg a : Outport  Port=7
  Mvg Avg b : Outport  Port=8
  Mvg Avg c : Outport  Port=9
  wires:
  Demux/1 -> V_a/1  "V_a"
  Demux/3 -> V_c/1  "V_c"
  Moving Variance1/1 -> Reshape1/1  "Mvg Var b"
  Moving Variance2/1 -> Reshape2/1  "Mvg Var c"
  Reshape/1 -> Mvg Var a/1  "Mvg Var a"
  Moving Average2/1 -> Reshape5/1  "Mvg Avg c"
  Demux2/3 -> Moving Average2/1
  Demux2/2 -> Moving Average1/1
  Moving Average/1 -> Reshape3/1  "Mvg Avg a"
  Demux11/3 -> Moving Variance2/1
  Demux11/1 -> Moving Variance/1
  Currents/1 -> Demux2/1, Demux11/1, Demux/1
  Moving Average1/1 -> Reshape4/1  "Mvg Avg b"
  Demux2/1 -> Moving Average/1
  Demux/2 -> V_b/1  "V_b"
  Demux11/2 -> Moving Variance1/1
  Moving Variance/1 -> Reshape/1
  Reshape1/1 -> Mvg Var b/1  "Mvg Var a"
  Reshape2/1 -> Mvg Var c/1  "Mvg Var a"
  Reshape3/1 -> Mvg Avg a/1  "Mvg Avg a"
  Reshape4/1 -> Mvg Avg b/1  "Mvg Avg b"
  Reshape5/1 -> Mvg Avg c/1  "Mvg Avg c"

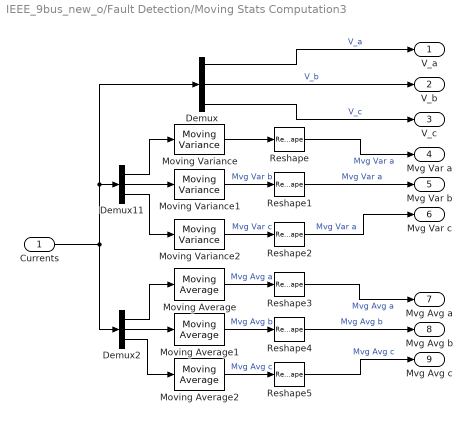
== system IEEE_9bus_new_o/Fault Detection/Moving Stats Computation3 ==
  Currents : Inport
  Demux : Demux  Outputs=3
  Demux11 : Demux  Outputs=3
  Demux2 : Demux  Outputs=3
  Moving Average : dspstat3/Moving Average  Method=Sliding window  ForgettingFactorPort=off  SpecifyWindowLength=on  WindowLength=100  OverlapLength=99  AllowArbitraryInputLength=off  ForgettingFactor=0.9  SimulateUsing=Interpreted execution
  Moving Average1 : dspstat3/Moving Average  Method=Sliding window  ForgettingFactorPort=off  SpecifyWindowLength=on  WindowLength=100  OverlapLength=99  AllowArbitraryInputLength=off  ForgettingFactor=0.9  SimulateUsing=Interpreted execution
  Moving Average2 : dspstat3/Moving Average  Method=Sliding window  ForgettingFactorPort=off  SpecifyWindowLength=on  WindowLength=100  OverlapLength=99  AllowArbitraryInputLength=off  ForgettingFactor=0.9  SimulateUsing=Interpreted execution
  Moving Variance : dspstat3/Moving Variance  Method=Sliding window  ForgettingFactorPort=off  SpecifyWindowLength=on  WindowLength=100  OverlapLength=99  AllowArbitraryInputLength=off  ForgettingFactor=0.9  SimulateUsing=Interpreted execution
  Moving Variance1 : dspstat3/Moving Variance  Method=Sliding window  ForgettingFactorPort=off  SpecifyWindowLength=on  WindowLength=100  OverlapLength=99  AllowArbitraryInputLength=off  ForgettingFactor=0.9  SimulateUsing=Interpreted execution
  Moving Variance2 : dspstat3/Moving Variance  Method=Sliding window  ForgettingFactorPort=off  SpecifyWindowLength=on  WindowLength=100  OverlapLength=99  AllowArbitraryInputLength=off  ForgettingFactor=0.9  SimulateUsing=Interpreted execution
  Reshape{,1..5} (6 alike) : Reshape  OutputDimensionality=Customize  OutputDimensions=1
  V_a : Outport
  V_b : Outport  Port=2
  V_c : Outport  Port=3
  Mvg Var a : Outport  Port=4
  Mvg Var b : Outport  Port=5
  Mvg Var c : Outport  Port=6
  Mvg Avg a : Outport  Port=7
  Mvg Avg b : Outport  Port=8
  Mvg Avg c : Outport  Port=9
  wires:
  Demux/1 -> V_a/1  "V_a"
  Demux/3 -> V_c/1  "V_c"
  Moving Variance1/1 -> Reshape1/1  "Mvg Var b"
  Moving Variance2/1 -> Reshape2/1  "Mvg Var c"
  Reshape/1 -> Mvg Var a/1  "Mvg Var a"
  Moving Average2/1 -> Reshape5/1  "Mvg Avg c"
  Demux2/3 -> Moving Average2/1
  Demux2/2 -> Moving Average1/1
  Moving Average/1 -> Reshape3/1  "Mvg Avg a"
  Demux11/3 -> Moving Variance2/1
  Demux11/1 -> Moving Variance/1
  Currents/1 -> Demux2/1, Demux11/1, Demux/1
  Moving Average1/1 -> Reshape4/1  "Mvg Avg b"
  Demux2/1 -> Moving Average/1
  Demux/2 -> V_b/1  "V_b"
  Demux11/2 -> Moving Variance1/1
  Moving Variance/1 -> Reshape/1
  Reshape1/1 -> Mvg Var b/1  "Mvg Var a"
  Reshape2/1 -> Mvg Var c/1  "Mvg Var a"
  Reshape3/1 -> Mvg Avg a/1  "Mvg Avg a"
  Reshape4/1 -> Mvg Avg b/1  "Mvg Avg b"
  Reshape5/1 -> Mvg Avg c/1  "Mvg Avg c"

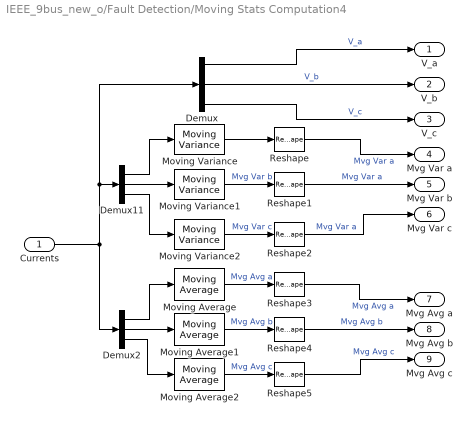
== system IEEE_9bus_new_o/Fault Detection/Moving Stats Computation4 ==
  Currents : Inport
  Demux : Demux  Outputs=3
  Demux11 : Demux  Outputs=3
  Demux2 : Demux  Outputs=3
  Moving Average : dspstat3/Moving Average  Method=Sliding window  ForgettingFactorPort=off  SpecifyWindowLength=on  WindowLength=100  OverlapLength=99  AllowArbitraryInputLength=off  ForgettingFactor=0.9  SimulateUsing=Interpreted execution
  Moving Average1 : dspstat3/Moving Average  Method=Sliding window  ForgettingFactorPort=off  SpecifyWindowLength=on  WindowLength=100  OverlapLength=99  AllowArbitraryInputLength=off  ForgettingFactor=0.9  SimulateUsing=Interpreted execution
  Moving Average2 : dspstat3/Moving Average  Method=Sliding window  ForgettingFactorPort=off  SpecifyWindowLength=on  WindowLength=100  OverlapLength=99  AllowArbitraryInputLength=off  ForgettingFactor=0.9  SimulateUsing=Interpreted execution
  Moving Variance : dspstat3/Moving Variance  Method=Sliding window  ForgettingFactorPort=off  SpecifyWindowLength=on  WindowLength=100  OverlapLength=99  AllowArbitraryInputLength=off  ForgettingFactor=0.9  SimulateUsing=Interpreted execution
  Moving Variance1 : dspstat3/Moving Variance  Method=Sliding window  ForgettingFactorPort=off  SpecifyWindowLength=on  WindowLength=100  OverlapLength=99  AllowArbitraryInputLength=off  ForgettingFactor=0.9  SimulateUsing=Interpreted execution
  Moving Variance2 : dspstat3/Moving Variance  Method=Sliding window  ForgettingFactorPort=off  SpecifyWindowLength=on  WindowLength=100  OverlapLength=99  AllowArbitraryInputLength=off  ForgettingFactor=0.9  SimulateUsing=Interpreted execution
  Reshape{,1..5} (6 alike) : Reshape  OutputDimensionality=Customize  OutputDimensions=1
  V_a : Outport
  V_b : Outport  Port=2
  V_c : Outport  Port=3
  Mvg Var a : Outport  Port=4
  Mvg Var b : Outport  Port=5
  Mvg Var c : Outport  Port=6
  Mvg Avg a : Outport  Port=7
  Mvg Avg b : Outport  Port=8
  Mvg Avg c : Outport  Port=9
  wires:
  Reshape5/1 -> Mvg Avg c/1  "Mvg Avg c"
  Reshape4/1 -> Mvg Avg b/1  "Mvg Avg b"
  Reshape3/1 -> Mvg Avg a/1  "Mvg Avg a"
  Reshape2/1 -> Mvg Var c/1  "Mvg Var a"
  Reshape1/1 -> Mvg Var b/1  "Mvg Var a"
  Moving Variance/1 -> Reshape/1
  Demux11/2 -> Moving Variance1/1
  Demux/2 -> V_b/1  "V_b"
  Demux2/1 -> Moving Average/1
  Moving Average1/1 -> Reshape4/1  "Mvg Avg b"
  Currents/1 -> Demux/1, Demux11/1, Demux2/1
  Demux11/1 -> Moving Variance/1
  Demux11/3 -> Moving Variance2/1
  Moving Average/1 -> Reshape3/1  "Mvg Avg a"
  Demux2/2 -> Moving Average1/1
  Demux2/3 -> Moving Average2/1
  Moving Average2/1 -> Reshape5/1  "Mvg Avg c"
  Reshape/1 -> Mvg Var a/1  "Mvg Var a"
  Moving Variance2/1 -> Reshape2/1  "Mvg Var c"
  Moving Variance1/1 -> Reshape1/1  "Mvg Var b"
  Demux/3 -> V_c/1  "V_c"
  Demux/1 -> V_a/1  "V_a"

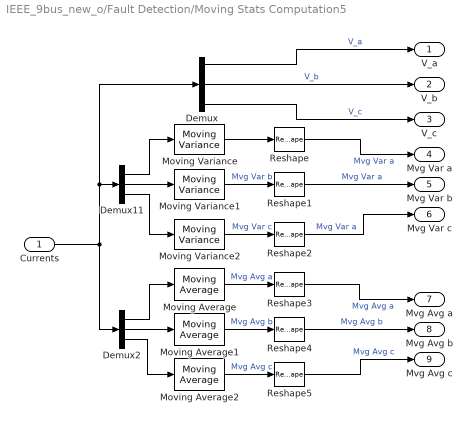
== system IEEE_9bus_new_o/Fault Detection/Moving Stats Computation5 ==
  Currents : Inport
  Demux : Demux  Outputs=3
  Demux11 : Demux  Outputs=3
  Demux2 : Demux  Outputs=3
  Moving Average : dspstat3/Moving Average  Method=Sliding window  ForgettingFactorPort=off  SpecifyWindowLength=on  WindowLength=100  OverlapLength=99  AllowArbitraryInputLength=off  ForgettingFactor=0.9  SimulateUsing=Interpreted execution
  Moving Average1 : dspstat3/Moving Average  Method=Sliding window  ForgettingFactorPort=off  SpecifyWindowLength=on  WindowLength=100  OverlapLength=99  AllowArbitraryInputLength=off  ForgettingFactor=0.9  SimulateUsing=Interpreted execution
  Moving Average2 : dspstat3/Moving Average  Method=Sliding window  ForgettingFactorPort=off  SpecifyWindowLength=on  WindowLength=100  OverlapLength=99  AllowArbitraryInputLength=off  ForgettingFactor=0.9  SimulateUsing=Interpreted execution
  Moving Variance : dspstat3/Moving Variance  Method=Sliding window  ForgettingFactorPort=off  SpecifyWindowLength=on  WindowLength=100  OverlapLength=99  AllowArbitraryInputLength=off  ForgettingFactor=0.9  SimulateUsing=Interpreted execution
  Moving Variance1 : dspstat3/Moving Variance  Method=Sliding window  ForgettingFactorPort=off  SpecifyWindowLength=on  WindowLength=100  OverlapLength=99  AllowArbitraryInputLength=off  ForgettingFactor=0.9  SimulateUsing=Interpreted execution
  Moving Variance2 : dspstat3/Moving Variance  Method=Sliding window  ForgettingFactorPort=off  SpecifyWindowLength=on  WindowLength=100  OverlapLength=99  AllowArbitraryInputLength=off  ForgettingFactor=0.9  SimulateUsing=Interpreted execution
  Reshape{,1..5} (6 alike) : Reshape  OutputDimensionality=Customize  OutputDimensions=1
  V_a : Outport
  V_b : Outport  Port=2
  V_c : Outport  Port=3
  Mvg Var a : Outport  Port=4
  Mvg Var b : Outport  Port=5
  Mvg Var c : Outport  Port=6
  Mvg Avg a : Outport  Port=7
  Mvg Avg b : Outport  Port=8
  Mvg Avg c : Outport  Port=9
  wires:
  Demux/1 -> V_a/1  "V_a"
  Demux/3 -> V_c/1  "V_c"
  Moving Variance1/1 -> Reshape1/1  "Mvg Var b"
  Moving Variance2/1 -> Reshape2/1  "Mvg Var c"
  Reshape/1 -> Mvg Var a/1  "Mvg Var a"
  Moving Average2/1 -> Reshape5/1  "Mvg Avg c"
  Demux2/3 -> Moving Average2/1
  Demux2/2 -> Moving Average1/1
  Moving Average/1 -> Reshape3/1  "Mvg Avg a"
  Demux11/3 -> Moving Variance2/1
  Demux11/1 -> Moving Variance/1
  Currents/1 -> Demux2/1, Demux11/1, Demux/1
  Moving Average1/1 -> Reshape4/1  "Mvg Avg b"
  Demux2/1 -> Moving Average/1
  Demux/2 -> V_b/1  "V_b"
  Demux11/2 -> Moving Variance1/1
  Moving Variance/1 -> Reshape/1
  Reshape1/1 -> Mvg Var b/1  "Mvg Var a"
  Reshape2/1 -> Mvg Var c/1  "Mvg Var a"
  Reshape3/1 -> Mvg Avg a/1  "Mvg Avg a"
  Reshape4/1 -> Mvg Avg b/1  "Mvg Avg b"
  Reshape5/1 -> Mvg Avg c/1  "Mvg Avg c"

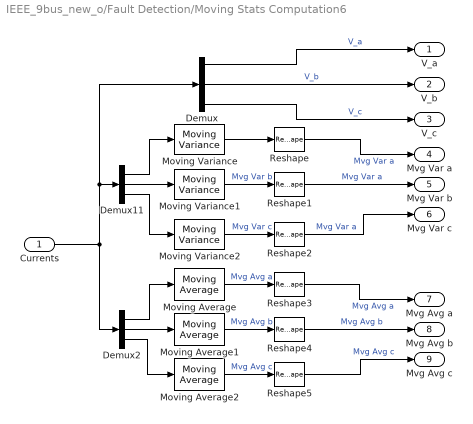
== system IEEE_9bus_new_o/Fault Detection/Moving Stats Computation6 ==
  Currents : Inport
  Demux : Demux  Outputs=3
  Demux11 : Demux  Outputs=3
  Demux2 : Demux  Outputs=3
  Moving Average : dspstat3/Moving Average  Method=Sliding window  ForgettingFactorPort=off  SpecifyWindowLength=on  WindowLength=100  OverlapLength=99  AllowArbitraryInputLength=off  ForgettingFactor=0.9  SimulateUsing=Interpreted execution
  Moving Average1 : dspstat3/Moving Average  Method=Sliding window  ForgettingFactorPort=off  SpecifyWindowLength=on  WindowLength=100  OverlapLength=99  AllowArbitraryInputLength=off  ForgettingFactor=0.9  SimulateUsing=Interpreted execution
  Moving Average2 : dspstat3/Moving Average  Method=Sliding window  ForgettingFactorPort=off  SpecifyWindowLength=on  WindowLength=100  OverlapLength=99  AllowArbitraryInputLength=off  ForgettingFactor=0.9  SimulateUsing=Interpreted execution
  Moving Variance : dspstat3/Moving Variance  Method=Sliding window  ForgettingFactorPort=off  SpecifyWindowLength=on  WindowLength=100  OverlapLength=99  AllowArbitraryInputLength=off  ForgettingFactor=0.9  SimulateUsing=Interpreted execution
  Moving Variance1 : dspstat3/Moving Variance  Method=Sliding window  ForgettingFactorPort=off  SpecifyWindowLength=on  WindowLength=100  OverlapLength=99  AllowArbitraryInputLength=off  ForgettingFactor=0.9  SimulateUsing=Interpreted execution
  Moving Variance2 : dspstat3/Moving Variance  Method=Sliding window  ForgettingFactorPort=off  SpecifyWindowLength=on  WindowLength=100  OverlapLength=99  AllowArbitraryInputLength=off  ForgettingFactor=0.9  SimulateUsing=Interpreted execution
  Reshape{,1..5} (6 alike) : Reshape  OutputDimensionality=Customize  OutputDimensions=1
  V_a : Outport
  V_b : Outport  Port=2
  V_c : Outport  Port=3
  Mvg Var a : Outport  Port=4
  Mvg Var b : Outport  Port=5
  Mvg Var c : Outport  Port=6
  Mvg Avg a : Outport  Port=7
  Mvg Avg b : Outport  Port=8
  Mvg Avg c : Outport  Port=9
  wires:
  Reshape5/1 -> Mvg Avg c/1  "Mvg Avg c"
  Reshape4/1 -> Mvg Avg b/1  "Mvg Avg b"
  Reshape3/1 -> Mvg Avg a/1  "Mvg Avg a"
  Reshape2/1 -> Mvg Var c/1  "Mvg Var a"
  Reshape1/1 -> Mvg Var b/1  "Mvg Var a"
  Moving Variance/1 -> Reshape/1
  Demux11/2 -> Moving Variance1/1
  Demux/2 -> V_b/1  "V_b"
  Demux2/1 -> Moving Average/1
  Moving Average1/1 -> Reshape4/1  "Mvg Avg b"
  Currents/1 -> Demux/1, Demux11/1, Demux2/1
  Demux11/1 -> Moving Variance/1
  Demux11/3 -> Moving Variance2/1
  Moving Average/1 -> Reshape3/1  "Mvg Avg a"
  Demux2/2 -> Moving Average1/1
  Demux2/3 -> Moving Average2/1
  Moving Average2/1 -> Reshape5/1  "Mvg Avg c"
  Reshape/1 -> Mvg Var a/1  "Mvg Var a"
  Moving Variance2/1 -> Reshape2/1  "Mvg Var c"
  Moving Variance1/1 -> Reshape1/1  "Mvg Var b"
  Demux/3 -> V_c/1  "V_c"
  Demux/1 -> V_a/1  "V_a"

== system IEEE_9bus_new_o/Fault Line Identification/If Action Subsystem ==
  In1 : Inport
  Action Port : ActionPort  ActionPortLabel=if(u1~=0)
  Out1 : Outport
  wires:
  In1/1 -> Out1/1

== system IEEE_9bus_new_o/Fault Line Identification/If Action Subsystem1 ==
  In1 : Inport
  Action Port : ActionPort  ActionPortLabel=else
  Out1 : Outport
  wires:
  In1/1 -> Out1/1

== system IEEE_9bus_new_o/Fault Location/If Action Subsystem ==
  In1 : Inport
  Action Port : ActionPort  ActionPortLabel=if(u1~=0)
  Out1 : Outport
  wires:
  In1/1 -> Out1/1

== system IEEE_9bus_new_o/Fault Location/If Action Subsystem1 ==
  In1 : Inport
  Action Port : ActionPort  ActionPortLabel=else
  Out1 : Outport
  wires:
  In1/1 -> Out1/1

== system IEEE_9bus_new_o/Fault Type Identification/If Action Subsystem ==
  In1 : Inport
  Action Port : ActionPort  ActionPortLabel=if(u1~=0)
  Out1 : Outport
  wires:
  In1/1 -> Out1/1

== system IEEE_9bus_new_o/Fault Type Identification/If Action Subsystem1 ==
  In1 : Inport
  Action Port : ActionPort  ActionPortLabel=else
  Out1 : Outport
  wires:
  In1/1 -> Out1/1

== system IEEE_9bus_new_o/Fault Detection/BUS Fault Detection1/Variance Threshold Computation ==
  Var : Inport
  Add Constant : Bias  Bias=-0.03  SaturateOnIntegerOverflow=off
  Clock : Clock
  Constant : Constant  Value=1/60
  Memory : Memory
  Relational Operator1 : RelationalOperator  Operator=<=  OutDataTypeStr=boolean  RndMeth=Simplest  InputSameDT=off
  Switch : Switch  Criteria=u2 > Threshold  SaturateOnIntegerOverflow=off  InputSameDT=off
  ThreshVar : Outport
  wires:
  Add Constant/1 -> ThreshVar/1  "Threshold var"
  Var/1 -> Switch/1
  Constant/1 -> Relational Operator1/2
  Relational Operator1/1 -> Switch/2
  Clock/1 -> Relational Operator1/1
  Switch/1 -> Memory/1, Add Constant/1  "BaseVar"
  Memory/1 -> Switch/3

== system IEEE_9bus_new_o/Fault Detection/BUS Fault Detection2/Variance Threshold Computation ==
  Var : Inport
  Add Constant : Bias  Bias=-0.03  SaturateOnIntegerOverflow=off
  Clock : Clock
  Constant : Constant  Value=1/60
  Memory : Memory
  Relational Operator1 : RelationalOperator  Operator=<=  OutDataTypeStr=boolean  RndMeth=Simplest  InputSameDT=off
  Switch : Switch  Criteria=u2 > Threshold  SaturateOnIntegerOverflow=off  InputSameDT=off
  ThreshVar : Outport
  wires:
  Memory/1 -> Switch/3
  Switch/1 -> Add Constant/1, Memory/1  "BaseVar"
  Clock/1 -> Relational Operator1/1
  Relational Operator1/1 -> Switch/2
  Constant/1 -> Relational Operator1/2
  Var/1 -> Switch/1
  Add Constant/1 -> ThreshVar/1  "Threshold var"

== system IEEE_9bus_new_o/Fault Detection/BUS Fault Detection3/Variance Threshold Computation ==
  Var : Inport
  Add Constant : Bias  Bias=-0.03  SaturateOnIntegerOverflow=off
  Clock : Clock
  Constant : Constant  Value=1/60
  Memory : Memory
  Relational Operator1 : RelationalOperator  Operator=<=  OutDataTypeStr=boolean  RndMeth=Simplest  InputSameDT=off
  Switch : Switch  Criteria=u2 > Threshold  SaturateOnIntegerOverflow=off  InputSameDT=off
  ThreshVar : Outport
  wires:
  Memory/1 -> Switch/3
  Switch/1 -> Add Constant/1, Memory/1  "BaseVar"
  Clock/1 -> Relational Operator1/1
  Relational Operator1/1 -> Switch/2
  Constant/1 -> Relational Operator1/2
  Var/1 -> Switch/1
  Add Constant/1 -> ThreshVar/1  "Threshold var"

== system IEEE_9bus_new_o/Fault Detection/BUS Fault Detection4/Variance Threshold Computation ==
  Var : Inport
  Add Constant : Bias  Bias=-0.03  SaturateOnIntegerOverflow=off
  Clock : Clock
  Constant : Constant  Value=1/60
  Memory : Memory
  Relational Operator1 : RelationalOperator  Operator=<=  OutDataTypeStr=boolean  RndMeth=Simplest  InputSameDT=off
  Switch : Switch  Criteria=u2 > Threshold  SaturateOnIntegerOverflow=off  InputSameDT=off
  ThreshVar : Outport
  wires:
  Add Constant/1 -> ThreshVar/1  "Threshold var"
  Var/1 -> Switch/1
  Constant/1 -> Relational Operator1/2
  Relational Operator1/1 -> Switch/2
  Clock/1 -> Relational Operator1/1
  Switch/1 -> Memory/1, Add Constant/1  "BaseVar"
  Memory/1 -> Switch/3

== system IEEE_9bus_new_o/Fault Detection/BUS Fault Detection5/Variance Threshold Computation ==
  Var : Inport
  Add Constant : Bias  Bias=-0.03  SaturateOnIntegerOverflow=off
  Clock : Clock
  Constant : Constant  Value=1/60
  Memory : Memory
  Relational Operator1 : RelationalOperator  Operator=<=  OutDataTypeStr=boolean  RndMeth=Simplest  InputSameDT=off
  Switch : Switch  Criteria=u2 > Threshold  SaturateOnIntegerOverflow=off  InputSameDT=off
  ThreshVar : Outport
  wires:
  Memory/1 -> Switch/3
  Switch/1 -> Add Constant/1, Memory/1  "BaseVar"
  Clock/1 -> Relational Operator1/1
  Relational Operator1/1 -> Switch/2
  Constant/1 -> Relational Operator1/2
  Var/1 -> Switch/1
  Add Constant/1 -> ThreshVar/1  "Threshold var"
